simulink model "idq"  (R2021a)
settings: Solver=VariableStepAuto  StartTime=0.0  StopTime=0.2  FixedStep=1/150000  MaxStep=1e-6
undefined symbols (not defined in the file): in, ou
libraries: neural x105, spsMosfetLib x12, simulink x5, pid_lib x3, spsabctodq0Lib x3, spsFirstOrderFilterLib x2, spsPermanentMagnetSynchronousMachineLib x2, spsCurrentMeasurementLib x2, spsDCVoltageSourceLib x2, spsThreePhaseVIMeasurementLib x2, spsabctoAlphaBetaZeroLib x2, spsSVPWMGenerator2LevelLib x1
(part 7 of 7)

== system idq/best iq/Layer 1/Delays 1 ==
  "p{1}" : Inport  PortDimensions=4  SampleTime=1e-05
      mask Display: e = 0.06;c1 = [120 230 180]/255;c2 = ([120 230 180]+0)/(256+128);c3 = ([120 230 180]+128)/(256+128);patch([0 1 1 0],[0 0 1 1],c1);patch([0 1 1 1-e 1-e 0+e],[0 0 1 1-e 0+e 0+e],c2);patch([0 0 1 1-e 0+e 0+e],[0 1 1 1-e 1-e 0+e],c3);plot([0 1 1 0 0],[0 0 1 1 0]);
  Delay 1 : UnitDelay  InitialCondition=pi_input_1_delayed_1  SampleTime=1e-05
      mask Display: e = 0.06;c1 = [120 150 230]/255;c2 = ([120 150 230]+0)/383;c3 = ([120 150 230]+128)/383;patch([0 1 1 0],[0 0 1 1],c1);patch([0 1 1 1-e 1-e 0+e],[0 0 1 1-e 0+e 0+e],c2);patch([0 0 1 1-e 0+e 0+e],[0 1 1 1-e 1-e 0+e],c3);plot([0 1 1 0 0],[0 0 1 1 0]);disp('D')
  Delay 2 : UnitDelay  InitialCondition=pi_input_1_delayed_2  SampleTime=1e-05
      mask Display: e = 0.06;c1 = [120 150 230]/255;c2 = ([120 150 230]+0)/383;c3 = ([120 150 230]+128)/383;patch([0 1 1 0],[0 0 1 1],c1);patch([0 1 1 1-e 1-e 0+e],[0 0 1 1-e 0+e 0+e],c2);patch([0 0 1 1-e 0+e 0+e],[0 1 1 1-e 1-e 0+e],c3);plot([0 1 1 0 0],[0 0 1 1 0]);disp('D')
  Delay 3 : UnitDelay  InitialCondition=pi_input_1_delayed_3  SampleTime=1e-05
      mask Display: e = 0.06;c1 = [120 150 230]/255;c2 = ([120 150 230]+0)/383;c3 = ([120 150 230]+128)/383;patch([0 1 1 0],[0 0 1 1],c1);patch([0 1 1 1-e 1-e 0+e],[0 0 1 1-e 0+e 0+e],c2);patch([0 0 1 1-e 0+e 0+e],[0 1 1 1-e 1-e 0+e],c3);plot([0 1 1 0 0],[0 0 1 1 0]);disp('D')
  Delay 4 : UnitDelay  InitialCondition=pi_input_1_delayed_4  SampleTime=1e-05
      mask Display: e = 0.06;c1 = [120 150 230]/255;c2 = ([120 150 230]+0)/383;c3 = ([120 150 230]+128)/383;patch([0 1 1 0],[0 0 1 1],c1);patch([0 1 1 1-e 1-e 0+e],[0 0 1 1-e 0+e 0+e],c2);patch([0 0 1 1-e 0+e 0+e],[0 1 1 1-e 1-e 0+e],c3);plot([0 1 1 0 0],[0 0 1 1 0]);disp('D')
  Delay 5 : UnitDelay  InitialCondition=pi_input_1_delayed_5  SampleTime=1e-05
      mask Display: e = 0.06;c1 = [120 150 230]/255;c2 = ([120 150 230]+0)/383;c3 = ([120 150 230]+128)/383;patch([0 1 1 0],[0 0 1 1],c1);patch([0 1 1 1-e 1-e 0+e],[0 0 1 1-e 0+e 0+e],c2);patch([0 0 1 1-e 0+e 0+e],[0 1 1 1-e 1-e 0+e],c3);plot([0 1 1 0 0],[0 0 1 1 0]);disp('D')
  mux : Mux  Inputs=5
      mask Display: e = 0.06;c1 = [120 150 230]/255;c2 = ([120 150 230]+0)/383;c3 = ([120 150 230]+128)/383;patch([0 1 1 0],[0 0 1 1],c1);patch([0 1 1 1-e 1-e 0+e],[0 0 1 1-e 0+e 0+e],c2);patch([0 0 1 1-e 0+e 0+e],[0 1 1 1-e 1-e 0+e],c3);plot([0 1 1 0 0],[0 0 1 1 0]);disp('Mux')
  "pd{1,1}" : Outport
      mask Display: e = 0.06;c1 = [120 230 180]/255;c2 = ([120 230 180]+0)/(256+128);c3 = ([120 230 180]+128)/(256+128);patch([0 1 1 0],[0 0 1 1],c1);patch([0 1 1 1-e 1-e 0+e],[0 0 1 1-e 0+e 0+e],c2);patch([0 0 1 1-e 0+e 0+e],[0 1 1 1-e 1-e 0+e],c3);plot([0 1 1 0 0],[0 0 1 1 0]);
  wires:
  "p{1}"/1 -> Delay 1/1
  Delay 1/1 -> Delay 2/1, mux/1
  Delay 2/1 -> Delay 3/1, mux/2
  Delay 3/1 -> Delay 4/1, mux/3
  Delay 4/1 -> Delay 5/1, mux/4
  Delay 5/1 -> mux/5
  mux/1 -> "pd{1,1}"/1

== system idq/best iq/Layer 1/Delays 2 ==
  "p{1}" : Inport  PortDimensions=1  SampleTime=1e-05
      mask Display: e = 0.06;c1 = [120 230 180]/255;c2 = ([120 230 180]+0)/(256+128);c3 = ([120 230 180]+128)/(256+128);patch([0 1 1 0],[0 0 1 1],c1);patch([0 1 1 1-e 1-e 0+e],[0 0 1 1-e 0+e 0+e],c2);patch([0 0 1 1-e 0+e 0+e],[0 1 1 1-e 1-e 0+e],c3);plot([0 1 1 0 0],[0 0 1 1 0]);
  Delay 1 : UnitDelay  InitialCondition=ai_layer_2_delayed_1  SampleTime=1e-05
      mask Display: e = 0.06;c1 = [120 150 230]/255;c2 = ([120 150 230]+0)/383;c3 = ([120 150 230]+128)/383;patch([0 1 1 0],[0 0 1 1],c1);patch([0 1 1 1-e 1-e 0+e],[0 0 1 1-e 0+e 0+e],c2);patch([0 0 1 1-e 0+e 0+e],[0 1 1 1-e 1-e 0+e],c3);plot([0 1 1 0 0],[0 0 1 1 0]);disp('D')
  Delay 2 : UnitDelay  InitialCondition=ai_layer_2_delayed_2  SampleTime=1e-05
      mask Display: e = 0.06;c1 = [120 150 230]/255;c2 = ([120 150 230]+0)/383;c3 = ([120 150 230]+128)/383;patch([0 1 1 0],[0 0 1 1],c1);patch([0 1 1 1-e 1-e 0+e],[0 0 1 1-e 0+e 0+e],c2);patch([0 0 1 1-e 0+e 0+e],[0 1 1 1-e 1-e 0+e],c3);plot([0 1 1 0 0],[0 0 1 1 0]);disp('D')
  Delay 3 : UnitDelay  InitialCondition=ai_layer_2_delayed_3  SampleTime=1e-05
      mask Display: e = 0.06;c1 = [120 150 230]/255;c2 = ([120 150 230]+0)/383;c3 = ([120 150 230]+128)/383;patch([0 1 1 0],[0 0 1 1],c1);patch([0 1 1 1-e 1-e 0+e],[0 0 1 1-e 0+e 0+e],c2);patch([0 0 1 1-e 0+e 0+e],[0 1 1 1-e 1-e 0+e],c3);plot([0 1 1 0 0],[0 0 1 1 0]);disp('D')
  Delay 4 : UnitDelay  InitialCondition=ai_layer_2_delayed_4  SampleTime=1e-05
      mask Display: e = 0.06;c1 = [120 150 230]/255;c2 = ([120 150 230]+0)/383;c3 = ([120 150 230]+128)/383;patch([0 1 1 0],[0 0 1 1],c1);patch([0 1 1 1-e 1-e 0+e],[0 0 1 1-e 0+e 0+e],c2);patch([0 0 1 1-e 0+e 0+e],[0 1 1 1-e 1-e 0+e],c3);plot([0 1 1 0 0],[0 0 1 1 0]);disp('D')
  Delay 5 : UnitDelay  InitialCondition=ai_layer_2_delayed_5  SampleTime=1e-05
      mask Display: e = 0.06;c1 = [120 150 230]/255;c2 = ([120 150 230]+0)/383;c3 = ([120 150 230]+128)/383;patch([0 1 1 0],[0 0 1 1],c1);patch([0 1 1 1-e 1-e 0+e],[0 0 1 1-e 0+e 0+e],c2);patch([0 0 1 1-e 0+e 0+e],[0 1 1 1-e 1-e 0+e],c3);plot([0 1 1 0 0],[0 0 1 1 0]);disp('D')
  mux : Mux  Inputs=5
      mask Display: e = 0.06;c1 = [120 150 230]/255;c2 = ([120 150 230]+0)/383;c3 = ([120 150 230]+128)/383;patch([0 1 1 0],[0 0 1 1],c1);patch([0 1 1 1-e 1-e 0+e],[0 0 1 1-e 0+e 0+e],c2);patch([0 0 1 1-e 0+e 0+e],[0 1 1 1-e 1-e 0+e],c3);plot([0 1 1 0 0],[0 0 1 1 0]);disp('Mux')
  "pd{1,2}" : Outport
      mask Display: e = 0.06;c1 = [120 230 180]/255;c2 = ([120 230 180]+0)/(256+128);c3 = ([120 230 180]+128)/(256+128);patch([0 1 1 0],[0 0 1 1],c1);patch([0 1 1 1-e 1-e 0+e],[0 0 1 1-e 0+e 0+e],c2);patch([0 0 1 1-e 0+e 0+e],[0 1 1 1-e 1-e 0+e],c3);plot([0 1 1 0 0],[0 0 1 1 0]);
  wires:
  "p{1}"/1 -> Delay 1/1
  Delay 1/1 -> Delay 2/1, mux/1
  Delay 2/1 -> Delay 3/1, mux/2
  Delay 3/1 -> Delay 4/1, mux/3
  Delay 4/1 -> Delay 5/1, mux/4
  Delay 5/1 -> mux/5
  mux/1 -> "pd{1,2}"/1

== system idq/best iq/Layer 1/IW{1,1} ==
  "pd{1,1}" : Inport  PortDimensions=20  SampleTime=1e-05
      mask Display: e = 0.06;c1 = [120 230 180]/255;c2 = ([120 230 180]+0)/(256+128);c3 = ([120 230 180]+128)/(256+128);patch([0 1 1 0],[0 0 1 1],c1);patch([0 1 1 1-e 1-e 0+e],[0 0 1 1-e 0+e 0+e],c2);patch([0 0 1 1-e 0+e 0+e],[0 1 1 1-e 1-e 0+e],c3);plot([0 1 1 0 0],[0 0 1 1 0]);
  "IW{1,1}(1,:)'" : Constant  Value=[-1.050815360146093890847396323806606233119964599609375;0.56128811122297339597508880615350790321826934814453125;-0.4603448404413039707350208118441514670848846435546875;2.42098690246052061780801523127593100070953369140625;1.0519222643419272600340264034457504749298095703125;-0.6907366532058019092943368377746082842350006103515625;-0.018972850464470385201121160889670136384665966033935546875;1.1763498727518537645408969183336012065410614013671875;0.34711736489120059712121246775495819747447967529296875;-0.2881324702984497942992447860888205468654632568359375;-0.191825652829712367530845540386508218944072723388671875;-0.034911025911158542756052014510714798234403133392333984375;-0.32860653567597741808725686496472917497158050537109375;0.06825811409812358732107639980313251726329326629638671875;-0.04077875210756597146311008827979094348847866058349609375;-1.4163428518763991892370768255204893648624420166015625;0.250371849425297610114427016014815308153629302978515625;-0.178201339427796534575776377096190117299556732177734375;0.5650609625612348363432602127431891858577728271484375;-1.8334439340373174243126186411245726048946380615234375]
      mask Display: e = 0.06;c1 = [120 150 230]/255;c2 = ([120 150 230]+0)/383;c3 = ([120 150 230]+128)/383;patch([0 1 1 0],[0 0 1 1],c1);patch([0 1 1 1-e 1-e 0+e],[0 0 1 1-e 0+e 0+e],c2);patch([0 0 1 1-e 0+e 0+e],[0 1 1 1-e 1-e 0+e],c3);plot([0 1 1 0 0],[0 0 1 1 0]);disp('Weights');
  "IW{1,1}(2,:)'" : Constant  Value=[-1.9753213613324926978265239085885696113109588623046875;-0.273077714484354305835012155512231402099132537841796875;-1.7819453736380677089101709498208947479724884033203125;0.587766167951282891834807742270641028881072998046875;1.9227868622497783501756885016220621764659881591796875;0.270813591961401811669674088989268057048320770263671875;-1.373749559830432342977246662485413253307342529296875;0.3016717237499559889357669817400164902210235595703125;0.6368885725709370060343417208059690892696380615234375;0.09815439784707265247210017378165503032505512237548828125;-0.46352128078867960159215044768643565475940704345703125;-0.0128413702451014265226714172740685171447694301605224609375;-0.922972428554441837178501373273320496082305908203125;-0.057092598327918249456747190606620279140770435333251953125;0.88475205832782066739383708409150131046772003173828125;-0.2616516877367776050533620946225710213184356689453125;0.60391216953795223698620020513772033154964447021484375;0.08276314355345955331433316359834861941635608673095703125;2.251209223249574176151099891285412013530731201171875;-0.453272205507715353345332687240443192422389984130859375]
      mask Display: e = 0.06;c1 = [120 150 230]/255;c2 = ([120 150 230]+0)/383;c3 = ([120 150 230]+128)/383;patch([0 1 1 0],[0 0 1 1],c1);patch([0 1 1 1-e 1-e 0+e],[0 0 1 1-e 0+e 0+e],c2);patch([0 0 1 1-e 0+e 0+e],[0 1 1 1-e 1-e 0+e],c3);plot([0 1 1 0 0],[0 0 1 1 0]);disp('Weights');
  "IW{1,1}(3,:)'" : Constant  Value=[-0.4762948825772654881660628234385512769222259521484375;-0.450725609474112831609460272375144995748996734619140625;-0.63514276825399296200203025364316999912261962890625;0.10126579234538470031257162418114603497087955474853515625;0.46712803461891072576150918393977917730808258056640625;0.42513176806661501228035149324568919837474822998046875;-0.494740122137905358190579363508732058107852935791015625;-0.49370683890203415078445914332405664026737213134765625;0.1538690465605720147923562990399659611284732818603515625;0.1502129474718522927911834585756878368556499481201171875;0.08293694087102469747474486894134315662086009979248046875;-0.228403488647438812630952043036813847720623016357421875;-0.2369371579803774829908746824003173969686031341552734375;-0.1597372046121410538166429660122958011925220489501953125;0.4140780735532418876942983843036927282810211181640625;-0.147170337081327262662711063967435620725154876708984375;0.1100508288467185735726161510683596134185791015625;0.143775976512600711654243923476315103471279144287109375;0.473824034118425718720146733176079578697681427001953125;0.72154378839899357966913839845801703631877899169921875]
      mask Display: e = 0.06;c1 = [120 150 230]/255;c2 = ([120 150 230]+0)/383;c3 = ([120 150 230]+128)/383;patch([0 1 1 0],[0 0 1 1],c1);patch([0 1 1 1-e 1-e 0+e],[0 0 1 1-e 0+e 0+e],c2);patch([0 0 1 1-e 0+e 0+e],[0 1 1 1-e 1-e 0+e],c3);plot([0 1 1 0 0],[0 0 1 1 0]);disp('Weights');
  "IW{1,1}(4,:)'" : Constant  Value=[1.59152443632813156426664136233739554882049560546875;1.2088047945522675252760791408945806324481964111328125;2.18348247771360615132607563282363116741180419921875;-0.2290906397562101071141427155453129671514034271240234375;-1.597675180341759482161023697699420154094696044921875;-1.1363086034320348804982359069981612265110015869140625;1.2269965332636301180713189751259051263332366943359375;-0.51899432429348835160709541014512069523334503173828125;-0.51961742938610466779891794431023299694061279296875;-0.350469470192787013740343127210508100688457489013671875;0.052448429767185500427473243689746595919132232666015625;-0.176737956923335548520270776862162165343761444091796875;0.61786392866640682530743333700229413807392120361328125;0.6768818840669743597260321621433831751346588134765625;-0.84739362693948450111491865754942409694194793701171875;0.1946507026218387836902223853030591271817684173583984375;-0.46514398340796692110643562045879662036895751953125;-0.327973385592520205733535476610995829105377197265625;-2.120868327844827039285746650421060621738433837890625;0.74002762577539271671156484444509260356426239013671875]
      mask Display: e = 0.06;c1 = [120 150 230]/255;c2 = ([120 150 230]+0)/383;c3 = ([120 150 230]+128)/383;patch([0 1 1 0],[0 0 1 1],c1);patch([0 1 1 1-e 1-e 0+e],[0 0 1 1-e 0+e 0+e],c2);patch([0 0 1 1-e 0+e 0+e],[0 1 1 1-e 1-e 0+e],c3);plot([0 1 1 0 0],[0 0 1 1 0]);disp('Weights');
  "IW{1,1}(5,:)'" : Constant  Value=[2.857058046316495847349870018661022186279296875;1.3951469877184792256485934558440931141376495361328125;4.29670542881071337859566483530215919017791748046875;-0.77986332015910264647828853412647731602191925048828125;-2.9342342739472027091096606454811990261077880859375;-1.3656628805677268889695596953970380127429962158203125;2.263029484570801219689428762649185955524444580078125;-0.37523073434166409612089410074986517429351806640625;-0.99083269114514960218542682923725806176662445068359375;-0.47130168246978187962525908005773089826107025146484375;0.0642387863847756757085250001182430423796176910400390625;0.02314173856928812555988628218983649276196956634521484375;1.2529502734520605589096930998493917286396026611328125;0.71302437836475274224312670412473380565643310546875;-2.232993517965493168730972683988511562347412109375;0.25289887656793996750792530292528681457042694091796875;-0.9007915817040605954701959490193985402584075927734375;-0.429012919874408538145615921166609041392803192138671875;-3.56019003408147138856065794243477284908294677734375;0.7944700530451040965118636449915356934070587158203125]
      mask Display: e = 0.06;c1 = [120 150 230]/255;c2 = ([120 150 230]+0)/383;c3 = ([120 150 230]+128)/383;patch([0 1 1 0],[0 0 1 1],c1);patch([0 1 1 1-e 1-e 0+e],[0 0 1 1-e 0+e 0+e],c2);patch([0 0 1 1-e 0+e 0+e],[0 1 1 1-e 1-e 0+e],c3);plot([0 1 1 0 0],[0 0 1 1 0]);disp('Weights');
  Mux : Mux  Inputs=5
      mask Display: e = 0.06;c1 = [120 150 230]/255;c2 = ([120 150 230]+0)/383;c3 = ([120 150 230]+128)/383;patch([0 1 1 0],[0 0 1 1],c1);patch([0 1 1 1-e 1-e 0+e],[0 0 1 1-e 0+e 0+e],c2);patch([0 0 1 1-e 0+e 0+e],[0 1 1 1-e 1-e 0+e],c3);plot([0 1 1 0 0],[0 0 1 1 0]);disp('Mux');
  dotprod{1..5} (5 alike) : neural/Weight Functions/dotprod
  "iz{1,1}" : Outport
      mask Display: e = 0.06;c1 = [120 230 180]/255;c2 = ([120 230 180]+0)/(256+128);c3 = ([120 230 180]+128)/(256+128);patch([0 1 1 0],[0 0 1 1],c1);patch([0 1 1 1-e 1-e 0+e],[0 0 1 1-e 0+e 0+e],c2);patch([0 0 1 1-e 0+e 0+e],[0 1 1 1-e 1-e 0+e],c3);plot([0 1 1 0 0],[0 0 1 1 0]);
  wires:
  "IW{1,1}(1,:)'"/1 -> dotprod1/1
  "pd{1,1}"/1 -> dotprod1/2, dotprod2/2, dotprod3/2, dotprod4/2, dotprod5/2
  dotprod1/1 -> Mux/1
  "IW{1,1}(2,:)'"/1 -> dotprod2/1
  dotprod2/1 -> Mux/2
  "IW{1,1}(3,:)'"/1 -> dotprod3/1
  dotprod3/1 -> Mux/3
  "IW{1,1}(4,:)'"/1 -> dotprod4/1
  dotprod4/1 -> Mux/4
  "IW{1,1}(5,:)'"/1 -> dotprod5/1
  dotprod5/1 -> Mux/5
  Mux/1 -> "iz{1,1}"/1

== system idq/best iq/Layer 1/LW{1,2} ==
  "ad{1,2}" : Inport  PortDimensions=5  SampleTime=1e-05
      mask Display: e = 0.06;c1 = [120 230 180]/255;c2 = ([120 230 180]+0)/(256+128);c3 = ([120 230 180]+128)/(256+128);patch([0 1 1 0],[0 0 1 1],c1);patch([0 1 1 1-e 1-e 0+e],[0 0 1 1-e 0+e 0+e],c2);patch([0 0 1 1-e 0+e 0+e],[0 1 1 1-e 1-e 0+e],c3);plot([0 1 1 0 0],[0 0 1 1 0]);
  "IW{1,2}(1,:)'" : Constant  Value=[-0.05343637584432571474568618441480793990194797515869140625;-0.13199192919497715337229237775318324565887451171875;0.133119918973663764472092907453770749270915985107421875;0.0308199967620364119469389407868220587261021137237548828125;-0.039255281710677845941059871393008506856858730316162109375]
      mask Display: e = 0.06;c1 = [120 150 230]/255;c2 = ([120 150 230]+0)/383;c3 = ([120 150 230]+128)/383;patch([0 1 1 0],[0 0 1 1],c1);patch([0 1 1 1-e 1-e 0+e],[0 0 1 1-e 0+e 0+e],c2);patch([0 0 1 1-e 0+e 0+e],[0 1 1 1-e 1-e 0+e],c3);plot([0 1 1 0 0],[0 0 1 1 0]);disp('weights');
  "IW{1,2}(2,:)'" : Constant  Value=[-0.032219850992390546007282381424374761991202831268310546875;-0.032029172529251991041743252708329237066209316253662109375;-0.031345339176573804029768410828182823024690151214599609375;0.09105363913225096583747841805234202183783054351806640625;-0.05655638272658812526483274041311233304440975189208984375]
      mask Display: e = 0.06;c1 = [120 150 230]/255;c2 = ([120 150 230]+0)/383;c3 = ([120 150 230]+128)/383;patch([0 1 1 0],[0 0 1 1],c1);patch([0 1 1 1-e 1-e 0+e],[0 0 1 1-e 0+e 0+e],c2);patch([0 0 1 1-e 0+e 0+e],[0 1 1 1-e 1-e 0+e],c3);plot([0 1 1 0 0],[0 0 1 1 0]);disp('weights');
  "IW{1,2}(3,:)'" : Constant  Value=[-0.0620479384739951733696017299735103733837604522705078125;-0.05203858709103241497739844589887070469558238983154296875;0.003847397818500017559195658378712323610670864582061767578125;0.061822708541771388690566624291022890247404575347900390625;-0.04246009469605231678723811228337581269443035125732421875]
      mask Display: e = 0.06;c1 = [120 150 230]/255;c2 = ([120 150 230]+0)/383;c3 = ([120 150 230]+128)/383;patch([0 1 1 0],[0 0 1 1],c1);patch([0 1 1 1-e 1-e 0+e],[0 0 1 1-e 0+e 0+e],c2);patch([0 0 1 1-e 0+e 0+e],[0 1 1 1-e 1-e 0+e],c3);plot([0 1 1 0 0],[0 0 1 1 0]);disp('weights');
  "IW{1,2}(4,:)'" : Constant  Value=[0.040437346994299995517341272943667718209326267242431640625;0.09468399899484424009354910367619595490396022796630859375;-0.05986965452284061239840440293846768327057361602783203125;-0.07549412733980000178579672365231090225279331207275390625;0.0618707113654987927997552787928725592792034149169921875]
      mask Display: e = 0.06;c1 = [120 150 230]/255;c2 = ([120 150 230]+0)/383;c3 = ([120 150 230]+128)/383;patch([0 1 1 0],[0 0 1 1],c1);patch([0 1 1 1-e 1-e 0+e],[0 0 1 1-e 0+e 0+e],c2);patch([0 0 1 1-e 0+e 0+e],[0 1 1 1-e 1-e 0+e],c3);plot([0 1 1 0 0],[0 0 1 1 0]);disp('weights');
  "IW{1,2}(5,:)'" : Constant  Value=[-0.00189462257343098639146561357193832009215839207172393798828125;0.06882947209682042932765710929743363521993160247802734375;0.0167175136308328996237460017937337397597730159759521484375;-0.10619214283333540393972072024553199298679828643798828125;0.08277493780584758986673676872669602744281291961669921875]
      mask Display: e = 0.06;c1 = [120 150 230]/255;c2 = ([120 150 230]+0)/383;c3 = ([120 150 230]+128)/383;patch([0 1 1 0],[0 0 1 1],c1);patch([0 1 1 1-e 1-e 0+e],[0 0 1 1-e 0+e 0+e],c2);patch([0 0 1 1-e 0+e 0+e],[0 1 1 1-e 1-e 0+e],c3);plot([0 1 1 0 0],[0 0 1 1 0]);disp('weights');
  Mux : Mux  Inputs=5
      mask Display: e = 0.06;c1 = [120 150 230]/255;c2 = ([120 150 230]+0)/383;c3 = ([120 150 230]+128)/383;patch([0 1 1 0],[0 0 1 1],c1);patch([0 1 1 1-e 1-e 0+e],[0 0 1 1-e 0+e 0+e],c2);patch([0 0 1 1-e 0+e 0+e],[0 1 1 1-e 1-e 0+e],c3);plot([0 1 1 0 0],[0 0 1 1 0]);disp('Mux');
  dotprod{1..5} (5 alike) : neural/Weight Functions/dotprod
  "lz{1,2}" : Outport
      mask Display: e = 0.06;c1 = [120 230 180]/255;c2 = ([120 230 180]+0)/(256+128);c3 = ([120 230 180]+128)/(256+128);patch([0 1 1 0],[0 0 1 1],c1);patch([0 1 1 1-e 1-e 0+e],[0 0 1 1-e 0+e 0+e],c2);patch([0 0 1 1-e 0+e 0+e],[0 1 1 1-e 1-e 0+e],c3);plot([0 1 1 0 0],[0 0 1 1 0]);
  wires:
  "IW{1,2}(1,:)'"/1 -> dotprod1/1
  "ad{1,2}"/1 -> dotprod1/2, dotprod2/2, dotprod3/2, dotprod4/2, dotprod5/2
  dotprod1/1 -> Mux/1
  "IW{1,2}(2,:)'"/1 -> dotprod2/1
  dotprod2/1 -> Mux/2
  "IW{1,2}(3,:)'"/1 -> dotprod3/1
  dotprod3/1 -> Mux/3
  "IW{1,2}(4,:)'"/1 -> dotprod4/1
  dotprod4/1 -> Mux/4
  "IW{1,2}(5,:)'"/1 -> dotprod5/1
  dotprod5/1 -> Mux/5
  Mux/1 -> "lz{1,2}"/1

== system idq/best iq/Layer 2/Delays 1 ==
  "p{2}" : Inport  PortDimensions=5  SampleTime=1e-05
      mask Display: e = 0.06;c1 = [120 230 180]/255;c2 = ([120 230 180]+0)/(256+128);c3 = ([120 230 180]+128)/(256+128);patch([0 1 1 0],[0 0 1 1],c1);patch([0 1 1 1-e 1-e 0+e],[0 0 1 1-e 0+e 0+e],c2);patch([0 0 1 1-e 0+e 0+e],[0 1 1 1-e 1-e 0+e],c3);plot([0 1 1 0 0],[0 0 1 1 0]);
  mux : Mux  Inputs=1
      mask Display: e = 0.06;c1 = [120 150 230]/255;c2 = ([120 150 230]+0)/383;c3 = ([120 150 230]+128)/383;patch([0 1 1 0],[0 0 1 1],c1);patch([0 1 1 1-e 1-e 0+e],[0 0 1 1-e 0+e 0+e],c2);patch([0 0 1 1-e 0+e 0+e],[0 1 1 1-e 1-e 0+e],c3);plot([0 1 1 0 0],[0 0 1 1 0]);disp('Mux')
  "pd{2,1}" : Outport
      mask Display: e = 0.06;c1 = [120 230 180]/255;c2 = ([120 230 180]+0)/(256+128);c3 = ([120 230 180]+128)/(256+128);patch([0 1 1 0],[0 0 1 1],c1);patch([0 1 1 1-e 1-e 0+e],[0 0 1 1-e 0+e 0+e],c2);patch([0 0 1 1-e 0+e 0+e],[0 1 1 1-e 1-e 0+e],c3);plot([0 1 1 0 0],[0 0 1 1 0]);
  wires:
  "p{2}"/1 -> mux/1
  mux/1 -> "pd{2,1}"/1

== system idq/best iq/Layer 2/LW{2,1} ==
  "ad{2,1}" : Inport  PortDimensions=5  SampleTime=1e-05
      mask Display: e = 0.06;c1 = [120 230 180]/255;c2 = ([120 230 180]+0)/(256+128);c3 = ([120 230 180]+128)/(256+128);patch([0 1 1 0],[0 0 1 1],c1);patch([0 1 1 1-e 1-e 0+e],[0 0 1 1-e 0+e 0+e],c2);patch([0 0 1 1-e 0+e 0+e],[0 1 1 1-e 1-e 0+e],c3);plot([0 1 1 0 0],[0 0 1 1 0]);
  "IW{2,1}(1,:)'" : Constant  Value=[-4.2441296656052234226308428333140909671783447265625;6.1132209714560357127766110352240502834320068359375;-11.8604520777037354406502345227636396884918212890625;-7.73936623620721775296260602772235870361328125;4.70888157485073666208563736290670931339263916015625]
      mask Display: e = 0.06;c1 = [120 150 230]/255;c2 = ([120 150 230]+0)/383;c3 = ([120 150 230]+128)/383;patch([0 1 1 0],[0 0 1 1],c1);patch([0 1 1 1-e 1-e 0+e],[0 0 1 1-e 0+e 0+e],c2);patch([0 0 1 1-e 0+e 0+e],[0 1 1 1-e 1-e 0+e],c3);plot([0 1 1 0 0],[0 0 1 1 0]);disp('weights');
  Mux : Mux  Inputs=1
      mask Display: e = 0.06;c1 = [120 150 230]/255;c2 = ([120 150 230]+0)/383;c3 = ([120 150 230]+128)/383;patch([0 1 1 0],[0 0 1 1],c1);patch([0 1 1 1-e 1-e 0+e],[0 0 1 1-e 0+e 0+e],c2);patch([0 0 1 1-e 0+e 0+e],[0 1 1 1-e 1-e 0+e],c3);plot([0 1 1 0 0],[0 0 1 1 0]);disp('Mux');
  dotprod1 : neural/Weight Functions/dotprod
  "lz{2,1}" : Outport
      mask Display: e = 0.06;c1 = [120 230 180]/255;c2 = ([120 230 180]+0)/(256+128);c3 = ([120 230 180]+128)/(256+128);patch([0 1 1 0],[0 0 1 1],c1);patch([0 1 1 1-e 1-e 0+e],[0 0 1 1-e 0+e 0+e],c2);patch([0 0 1 1-e 0+e 0+e],[0 1 1 1-e 1-e 0+e],c3);plot([0 1 1 0 0],[0 0 1 1 0]);
  wires:
  "IW{2,1}(1,:)'"/1 -> dotprod1/1
  "ad{2,1}"/1 -> dotprod1/2
  dotprod1/1 -> Mux/1
  Mux/1 -> "lz{2,1}"/1

== matlab function idq/MATLAB Function1 ==
  data: i input; u input; y output
function y = fcn(i, u)
    
y = u(i+1,:);

== matlab function idq/MATLAB Function ==
  data: u input; y output
function y = fcn(u)
    u = u - (2*pi*floor(u/(2*pi)));
y = u;

== matlab function idq/Triggered Subsystem/MATLAB Function2 ==
  data: we input; id input; iq input; iqref input; ang input; d output; angle output; vsq output; vq input
function [d,angle,vsq]  = MPC(we,id,iq,iqref,ang, vq)

persistent oldState c;

if isempty(oldState)
    oldState = 1;
    psiq = 0;
    c  = 1;
end
b = 0;
Ts = 1/40000;
Vdc = 12;
L = 2*0.0004;
R = 2*0.75 + 2*0.052;
psiPM = 0.00666;

p = 0.5;
q = 0.5;
r = 0.25;
s = 0.0;

states = [1 0    0 1    0 1;
         1 0    1 0    0 1;
         0 1    1 0    0 1;
         0 1    1 0    1 0;
         0 1    0 1    1 0;
         1 0    0 1    1 0;
         0 1    0 1    0 1;
         1 0    1 0    1 0];

y = states(1,:)';
cost = [];

for i=1:length(states)
    Sa=states(i,1);
    Sb=states(i,3);
    Sc=states(i,5);
    
    Va=(Vdc*(2*Sa-Sb-Sc))/3;
    Vb=(Vdc*(2*Sb-Sa-Sc))/3;
    Vc=(Vdc*(2*Sc-Sb-Sa))/3;
    
    vsd = (2/3)*[sin(ang) sin(ang - (2*pi/3)) sin(ang + (2*pi/3))]*[Va Vb Vc]';
    vsq = (2/3)*[cos(ang) cos(ang - (2*pi/3)) cos(ang + (2*pi/3))]*[Va Vb Vc]';

    
    m = ~(states(i,:) == states(oldState,:));
    
    id_p = id;
    iq_p = iq;
    
    cTemp = 0;
    for x = 1:3
        xx = ((1-(R*Ts/L))*id_p)+(Ts*we*iq_p)+(vsd*Ts/L);
        yy = ((1-(R*Ts/L))*iq_p)-(Ts*we*id_p)-(psiPM*we*Ts/L)+(vsq*Ts/L);
    
        id_p = xx;
        iq_p = yy;
        
        ia = cos(ang)*id_p - sin(ang)*iq_p;
        ib = cos(ang - (2*pi/3))*id_p - sin(ang - (2*pi/3))*iq_p;
        ic = cos(ang + (2*pi/3))*id_p - sin(ang + (2*pi/3))*iq_p;

        if abs(iq_p) > 3
            cTemp = cTemp + 1000*(abs(iq_p) - 3)^2;
        end
        
        mosfetLoss = 0;
        cTemp = cTemp + 0.1*(0 - id_p)^2 + (iqref - iq_p)^2;
    end
    

    cost = [cost  cTemp]
end

a = find(cost == min(cost));
a = a(end);
% if(abs(cost(a) - cost(oldState)) < 0.1)
%    a = oldState;
% end


if(a ~= oldState)
    c = c+1;
    
    if(a == 7 || a == 8)
       if(oldState == 1 || oldState == 3 || oldState == 5 || oldState == 8)
          a = 8; 
       elseif(oldState == 2 || oldState == 4 || oldState == 6 || oldState == 7)
           a = 7;
       end
    end
    
    oldState = a;
end
d=c;

b = vsq;

% angle = (a-1)*pi/3;
angle = states(a,:);

== matlab function idq/MATLAB Function2 ==
  data: i input; u input; y output
function y = fcn(i, u)
    
y = u(i+1,:);

== matlab function idq/MATLAB Function5 ==
  data: u input; y output
function y= fcn(u)
    u = (u+0.5)*2*pi;
y = u;
